simulink model "BSD_System"  (R2024a)
settings: Solver=FixedStepDiscrete  StartTime=0.0  StopTime=10  FixedStep=0.02  RelTol=1e-3
settings Model: Creator=pc  LastModifiedBy=pc
settings OptimizationCC: DefaultParameterBehavior=Inlined  EnhancedBackFolding=on  PassReuseOutputArgsAs=Individual arguments  ZeroExternalMemoryAtStartup=off  ZeroInternalMemoryAtStartup=off  OptimizeBlockOrder=speed  DifferentSizesBufferReuse=on  OptimizationCustomize=off  EfficientTunableParamExpr=on
settings DebuggingCC: ParameterTunabilityLossMsg=error
settings SFSimCC: MATLABDynamicMemAlloc=off
settings RTWCC: Description=AUTOSAR  SystemTargetFile=autosar.tlc  GenCodeOnly=on  TemplateMakefile=ert_default_tmf  GenerateReport=on  BuildConfiguration=Faster Runs  LaunchReport=on  DataTypeReplacement=CDataTypesFixedWidth
settings CodeAppCC: ForceParamTrailComments=on  IgnoreCustomStorageClasses=off  OperatorAnnotations=on  SimulinkDataObjDesc=on  SFDataObjDesc=on  InsertBlockDesc=on
settings STFCustomTargetCC: MultiwordLength=256  ParMdlRefBuildCompliant=on  CompOptLevelCompliant=on  IncludeMdlTerminateFcn=off  CombineOutputUpdateFcns=on  SuppressErrorStatus=on  ERTCustomFileBanners=on  SupportNonFinite=off  SupportComplex=off  SupportContinuousTime=off  SupportNonInlinedSFcns=off  RemoveResetFunc=on  MATLABClassNameForMDSCustomization=Simulink.SoftwareTarget.ERTCustomization  AutosarCompliant=on  GRTInterface=off  LookupTableObjectStructAxisOrder=2,1,3,4,...  LUTObjectStructOrderEvenSpacing=Size,Table,Breakpoints  SystemTargetFile=autosar.tlc
settings ERTTargetCC: TargetLangStandard=C99 (ISO)  ConcurrentExecutionCompliant=off  IncludeMdlTerminateFcn=off  SuppressErrorStatus=on  SupportNonFinite=off  SupportComplex=off  ModelStepFunctionPrototypeControlCompliant=off  CPPClassGenCompliant=off  AutosarCompliant=on  LookupTableObjectStructAxisOrder=2,1,3,4,...  LUTObjectStructOrderEvenSpacing=Size,Table,Breakpoints  InlinedParameterPlacement=NonHierarchical  ERTCustomFileTemplate=example_file_process.tlc  BooleanTrueId=TRUE  BooleanFalseId=FALSE

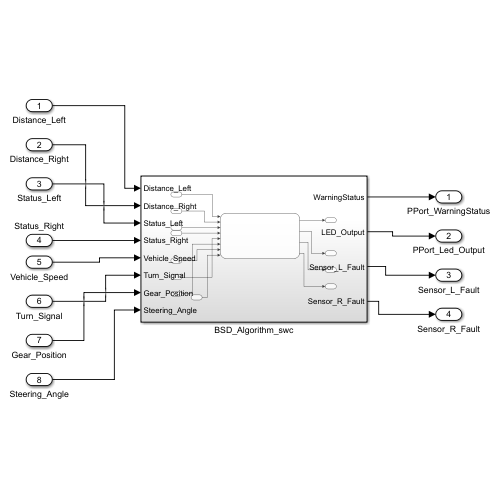
[thumbnail: Simulink's stored preview of the top-level diagram]
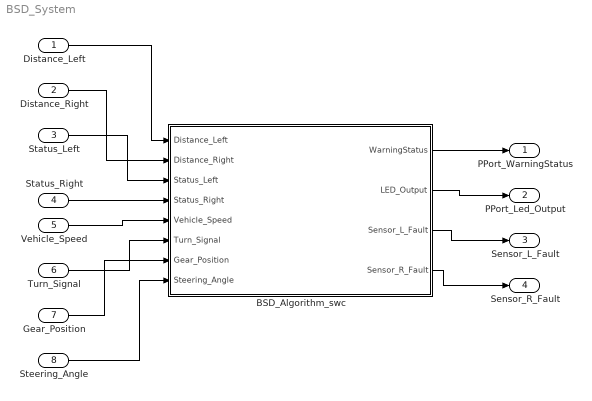
== system BSD_System ==
  Distance_Left : Inport
  Distance_Right : Inport  Port=2
  Status_Left : Inport  Port=3
  Status_Right : Inport  Port=4
  Vehicle_Speed : Inport  Port=5  OutDataTypeStr=single
  Turn_Signal : Inport  Port=6  OutDataTypeStr=uint8
  Gear_Position : Inport  Port=7  OutDataTypeStr=uint8
  Steering_Angle : Inport  Port=8  OutDataTypeStr=single
  BSD_Algorithm_swc : Subsystem
  PPort_WarningStatus : Outport
  PPort_Led_Output : Outport  Port=2
  Sensor_L_Fault : Outport  Port=3
  Sensor_R_Fault : Outport  Port=4
  wires:
  Distance_Left/1 -> BSD_Algorithm_swc/1(Distance_Left)
  Distance_Right/1 -> BSD_Algorithm_swc/2(Distance_Right)
  Status_Left/1 -> BSD_Algorithm_swc/3(Status_Left)
  Status_Right/1 -> BSD_Algorithm_swc/4(Status_Right)
  Vehicle_Speed/1 -> BSD_Algorithm_swc/5(Vehicle_Speed)
  Turn_Signal/1 -> BSD_Algorithm_swc/6(Turn_Signal)
  Gear_Position/1 -> BSD_Algorithm_swc/7(Gear_Position)
  Steering_Angle/1 -> BSD_Algorithm_swc/8(Steering_Angle)
  BSD_Algorithm_swc/3(Sensor_L_Fault) -> Sensor_L_Fault/1
  BSD_Algorithm_swc/1(WarningStatus) -> PPort_WarningStatus/1
  BSD_Algorithm_swc/4(Sensor_R_Fault) -> Sensor_R_Fault/1
  BSD_Algorithm_swc/2(LED_Output) -> PPort_Led_Output/1

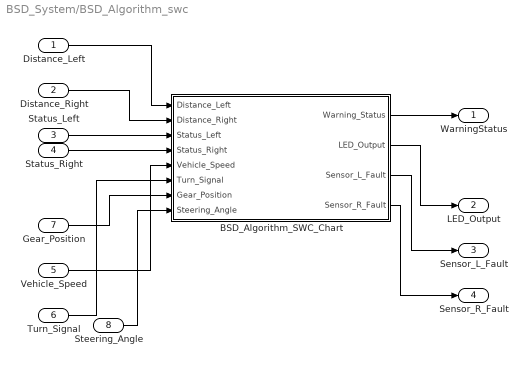
== system BSD_System/BSD_Algorithm_swc ==
  Distance_Left : Inport  OutDataTypeStr=single  Unit=m
  Distance_Right : Inport  Port=2  OutDataTypeStr=single
  Status_Left : Inport  Port=3  OutDataTypeStr=uint8
  Status_Right : Inport  Port=4  OutDataTypeStr=uint8
  Vehicle_Speed : Inport  Port=5  OutDataTypeStr=single  Unit=km/h
  Turn_Signal : Inport  Port=6  OutDataTypeStr=uint8
  Gear_Position : Inport  Port=7  OutDataTypeStr=uint8
  Steering_Angle : Inport  Port=8  OutDataTypeStr=single
  BSD_Algorithm_SWC_Chart : Stateflow chart  TreatAsAtomicUnit=on
  WarningStatus : Outport  OutDataTypeStr=uint8
  LED_Output : Outport  Port=2  OutDataTypeStr=uint8
  Sensor_L_Fault : Outport  Port=3  OutDataTypeStr=uint8
  Sensor_R_Fault : Outport  Port=4  OutDataTypeStr=uint8
  wires:
  Distance_Left/1 -> BSD_Algorithm_SWC_Chart/1(Distance_Left)
  Vehicle_Speed/1 -> BSD_Algorithm_SWC_Chart/5(Vehicle_Speed)
  Turn_Signal/1 -> BSD_Algorithm_SWC_Chart/6(Turn_Signal)
  Status_Right/1 -> BSD_Algorithm_SWC_Chart/4(Status_Right)
  Gear_Position/1 -> BSD_Algorithm_SWC_Chart/7(Gear_Position)
  Distance_Right/1 -> BSD_Algorithm_SWC_Chart/2(Distance_Right)
  BSD_Algorithm_SWC_Chart/1(Warning_Status) -> WarningStatus/1
  Status_Left/1 -> BSD_Algorithm_SWC_Chart/3(Status_Left)
  BSD_Algorithm_SWC_Chart/2(LED_Output) -> LED_Output/1
  BSD_Algorithm_SWC_Chart/3(Sensor_L_Fault) -> Sensor_L_Fault/1
  BSD_Algorithm_SWC_Chart/4(Sensor_R_Fault) -> Sensor_R_Fault/1
  Steering_Angle/1 -> BSD_Algorithm_SWC_Chart/8(Steering_Angle)

== stateflow chart BSD_System/BSD_Algorithm_swc/BSD_Algorithm_SWC_Chart ==
  state CLEAR
    entry:
    Warning_Status = uint8(0);
    LED_Output       = uint8(0);
    du:
    %% Fault detection
    Sensor_L_Fault = uint8(Status_Left  ~= uint8(0));
    Sensor_R_Fault = uint8(Status_Right ~= uint8(0));
    %% Effective distance calculation
    if (Status_Left ~= uint8(0)) && (Status_Right ~= uint8(0))
    effective_dist = single(99.0);
    elseif Status_Left ~= uint8(0)
    effective_dist = Distance_Right;
    elseif Status_Right ~= uint8(0)
    effective_dist = Distance_Left;
    else
    effective_dist = min(Distance_Left, Distance_Right);
    end
  state WARNING
    entry:
    Warning_Status = uint8(1);
    LED_Output      = uint8(1);
    du:
    %% Fault detection
    Sensor_L_Fault = uint8(Status_Left  ~= uint8(0));
    Sensor_R_Fault = uint8(Status_Right ~= uint8(0));
    %% Effective distance calculation
    if (Status_Left ~= uint8(0)) && (Status_Right ~= uint8(0))
    effective_dist = single(99.0);
    elseif Status_Left ~= uint8(0)
    effective_dist = Distance_Right;
    elseif Status_Right ~= uint8(0)
    effective_dist = Distance_Left;
    else
    effective_dist = min(Distance_Left, Distance_Right);
    end
  state ALERT
    entry:
    Warning_Status = uint8(2);
    LED_Output      = uint8(1);
    du:
    %% Fault detection
    Sensor_L_Fault = uint8(Status_Left  ~= uint8(0));
    Sensor_R_Fault = uint8(Status_Right ~= uint8(0));
    %% Effective distance calculation
    if (Status_Left ~= uint8(0)) && (Status_Right ~= uint8(0))
    effective_dist = single(99.0);
    elseif Status_Left ~= uint8(0)
    effective_dist = Distance_Right;
    elseif Status_Right ~= uint8(0)
    effective_dist = Distance_Left;
    else
    effective_dist = min(Distance_Left, Distance_Right);
    end
  (default) -> CLEAR
  CLEAR -> WARNING : [effective_dist < single(3.0) && Vehicle_Speed  > single(10.0) && Gear_Position  == uint8(3)&& abs(Steering_Angle) < single(45.0)]
  WARNING -> CLEAR [order 1] : [effective_dist >= single(3.0) ||  Vehicle_Speed  <= single(10.0) ||  Gear_Position  ~= uint8(3)|| abs(Steering_Angle) >= single(45.0)]
  ALERT -> WARNING [order 1] : [Turn_Signal == 0 && abs(Steering_Angle) <= single(15.0)]
  WARNING -> ALERT [order 2] : [effective_dist < single(3.0) &&  Vehicle_Speed  > single(10.0) &&  Turn_Signal > uint8(0) && abs(Steering_Angle) > single(15.0)]
  ALERT -> CLEAR [order 2] : [effective_dist >= single(3.0) ||  Vehicle_Speed  <= single(10.0) ||  Gear_Position  ~= uint8(3)]
  data: Distance_Left input single; Distance_Right input single; Status_Left input uint8; Status_Right input uint8; Vehicle_Speed input single; Turn_Signal input uint8; Gear_Position input uint8; Warning_Status output uint8; LED_Output output uint8; Sensor_L_Fault output uint8; Sensor_R_Fault output uint8; effective_dist local single =99.0; Steering_Angle input single
